simulink model "Sim_Ex32"  (R2022a)
settings: Solver=VariableStepAuto  StartTime=0.0  StopTime=Stop_Time  MaxStep=100e-6  RelTol=1e-3
values from neighbouring files (symbols this model uses):
  Ts = 1/Fs    (= 5e-05)    [A_Ex32.m]
undefined symbols (not defined in the file or in its folder): DiscIntNeverNeededParam, Grid, PLL
settings Model: SimulationMode=accelerator  Creator=Joonhee  LastModifiedBy=light
settings SolverCC: AlgebraicLoopSolver=TrustRegion
settings DataIOCC: ReturnWorkspaceOutputs=off
settings DebuggingCC: UnconnectedInputMsg=warning  UnconnectedOutputMsg=warning  UnconnectedLineMsg=warning  SFMachineParentedDataDiag=warning  ArithmeticOperatorsInVariantConditions=warning
settings SFSimCC: SimUseLocalCustomCode=off  CustomCodeUndefinedFunction=UseInterfaceOnly
settings RTWCC: RTWUseLocalCustomCode=off
settings CodeAppCC: StateflowObjectComments=on

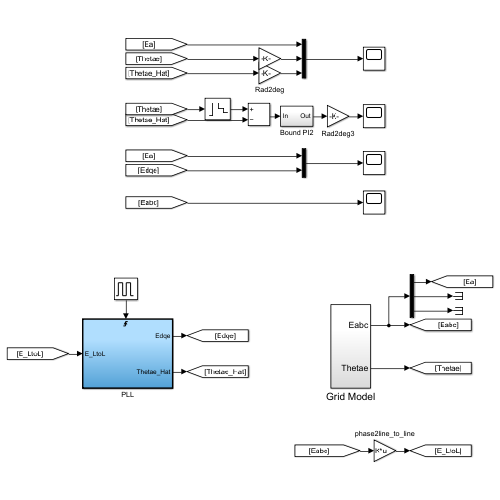
[thumbnail: Simulink's stored preview of the top-level diagram]
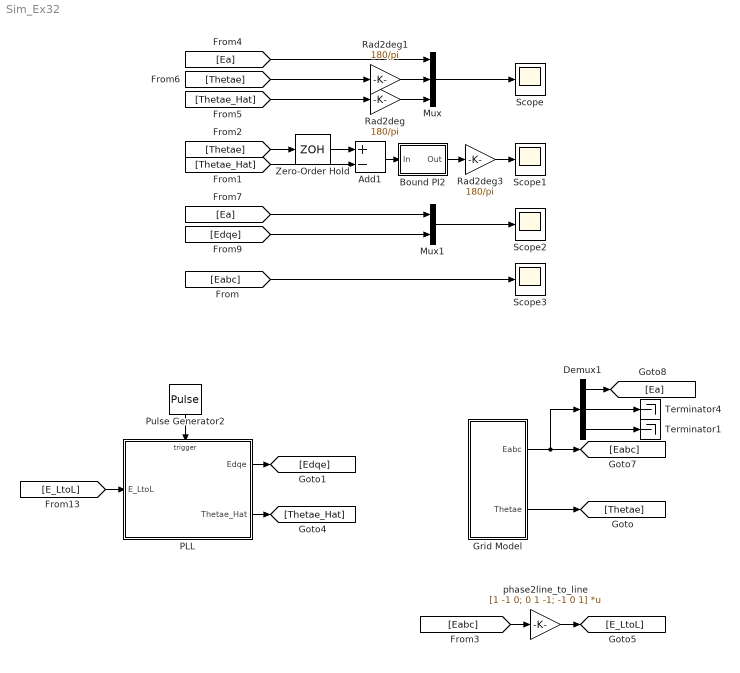
== system Sim_Ex32 ==
  Add1 : Sum  Inputs=+-
  Bound PI2 : Subsystem
  Demux1 : Demux  Outputs=3
  Grid Model : Subsystem
  Mux : Mux  Inputs=3
  Mux1 : Mux  Inputs=2
  PLL : Subsystem  TreatAsAtomicUnit=on
  Pulse Generator2 : DiscretePulseGenerator  PulseType=Time based  Period=Ts  PulseWidth=50
  Rad2deg : Gain  Gain=180/pi
  Rad2deg1 : Gain  Gain=180/pi
  Rad2deg3 : Gain  Gain=180/pi
  Scope{,1..3} (4 alike) : Scope
  Terminator1 : Terminator
  Terminator4 : Terminator
  Zero-Order Hold : ZeroOrderHold  SampleTime=Ts
  phase2line_to_line : Gain  Gain=[1 -1 0; 0 1 -1; -1 0 1]  Multiplication=Matrix(K*u)
  wires:
  Mux/1 -> Scope/1
  [Thetae_Hat] -> Rad2deg/1
  Rad2deg/1 -> Mux/3
  [Thetae] -> Rad2deg1/1
  Rad2deg1/1 -> Mux/2
  [Ea] -> Mux/1
  Mux1/1 -> Scope2/1
  [Ea] -> Mux1/1
  [Edqe] -> Mux1/2
  PLL/2(Thetae_Hat) -> [Thetae_Hat]
  PLL/1(Edqe) -> [Edqe]
  Pulse Generator2/1 -> PLL/Trigger
  Rad2deg3/1 -> Scope1/1
  Add1/1 -> Bound PI2/1(In)
  [Thetae_Hat] -> Add1/2
  Bound PI2/1(Out) -> Rad2deg3/1
  [Thetae] -> Zero-Order Hold/1
  Zero-Order Hold/1 -> Add1/1
  [Eabc] -> Scope3/1
  Demux1/1 -> [Ea]
  Demux1/2 -> Terminator4/1
  Demux1/3 -> Terminator1/1
  phase2line_to_line/1 -> [E_LtoL]
  [Eabc] -> phase2line_to_line/1
  [E_LtoL] -> PLL/1(E_LtoL)
  Grid Model/1(Eabc) -> Demux1/1, [Eabc]
  Grid Model/2(Thetae) -> [Thetae]

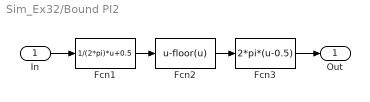
== system Sim_Ex32/Bound PI2 ==
  In : Inport
  Fcn1 : Fcn  Expr=1/(2*pi)*u+0.5
  Fcn2 : Fcn  Expr=u-floor(u)
  Fcn3 : Fcn  Expr=2*pi*(u-0.5)
  Out : Outport
  wires:
  Fcn1/1 -> Fcn2/1
  Fcn2/1 -> Fcn3/1
  In/1 -> Fcn1/1
  Fcn3/1 -> Out/1

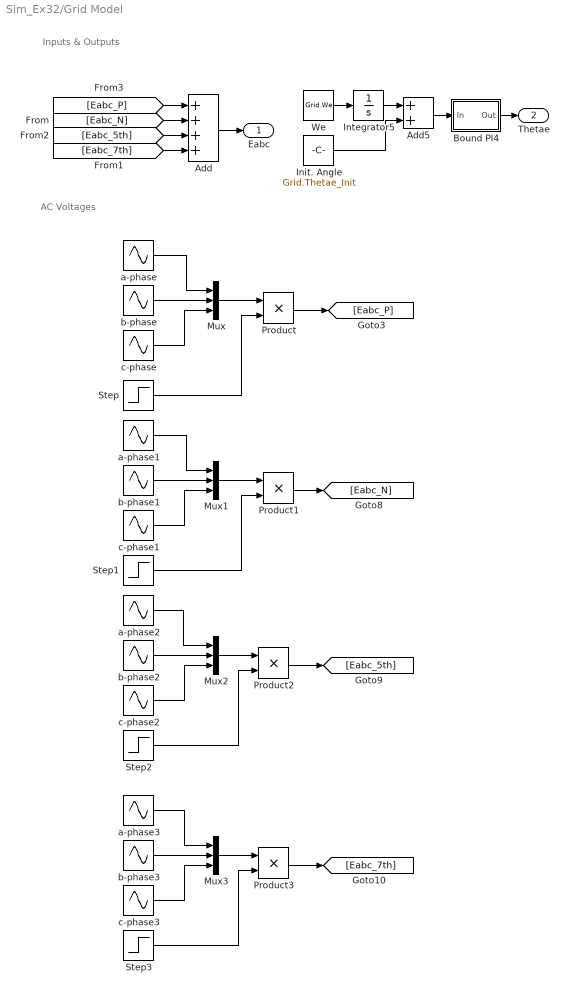
== system Sim_Ex32/Grid Model ==
  note: AC Voltages
  note: Inputs & Outputs
  Add : Sum  Inputs=++++
  Add5 : Sum
  Bound PI4 : Subsystem
  Init. Angle : Constant  Value=Grid.Thetae_Init
  Integrator5 : Integrator
  Mux{,1..3} (4 alike) : Mux  Inputs=3
  Product{,1..3} (4 alike) : Product
  Step : Step  Time=Grid.Time_Fault  Before=1  After=Grid.Ratio_P  SampleTime=0
  Step1 : Step  Time=Grid.Time_Fault  SampleTime=0
  Step2 : Step  Time=Grid.Time_Fault  SampleTime=0
  Step3 : Step  Time=Grid.Time_Fault  SampleTime=0
  We : Constant  Value=Grid.We
  a-phase : Sin  Amplitude=Grid.V_P  Frequency=Grid.We  Phase=Grid.Thetae_Init+pi  SampleTime=0
  a-phase1 : Sin  Amplitude=Grid.V_N  Frequency=Grid.We  Phase=Grid.Thetae_N_Init+pi  SampleTime=0
  a-phase2 : Sin  Amplitude=Grid.V_5th  Frequency=5*Grid.We  Phase=Grid.Thetae_5th_Init+pi  SampleTime=0
  a-phase3 : Sin  Amplitude=Grid.V_7th  Frequency=7*Grid.We  Phase=Grid.Thetae_7th_Init+pi  SampleTime=0
  b-phase : Sin  Amplitude=Grid.V_P  Frequency=Grid.We  Phase=Grid.Thetae_Init+pi-2/3*pi  SampleTime=0
  b-phase1 : Sin  Amplitude=Grid.V_N  Frequency=Grid.We  Phase=Grid.Thetae_N_Init+pi+2/3*pi  SampleTime=0
  b-phase2 : Sin  Amplitude=Grid.V_5th  Frequency=5*Grid.We  Phase=Grid.Thetae_5th_Init+pi+2/3*pi  SampleTime=0
  b-phase3 : Sin  Amplitude=Grid.V_7th  Frequency=7*Grid.We  Phase=Grid.Thetae_7th_Init+pi-2/3*pi  SampleTime=0
  c-phase : Sin  Amplitude=Grid.V_P  Frequency=Grid.We  Phase=Grid.Thetae_Init+pi-4/3*pi  SampleTime=0
  c-phase1 : Sin  Amplitude=Grid.V_N  Frequency=Grid.We  Phase=Grid.Thetae_N_Init+pi+4/3*pi  SampleTime=0
  c-phase2 : Sin  Amplitude=Grid.V_5th  Frequency=5*Grid.We  Phase=Grid.Thetae_5th_Init+pi+4/3*pi  SampleTime=0
  c-phase3 : Sin  Amplitude=Grid.V_7th  Frequency=7*Grid.We  Phase=Grid.Thetae_7th_Init+pi-4/3*pi  SampleTime=0
  Eabc : Outport
  Thetae : Outport  Port=2
  wires:
  [Eabc_P] -> Add/1
  Add/1 -> Eabc/1
  [Eabc_N] -> Add/2
  [Eabc_5th] -> Add/3
  [Eabc_7th] -> Add/4
  Bound PI4/1(Out) -> Thetae/1
  Add5/1 -> Bound PI4/1(In)
  We/1 -> Integrator5/1
  Init. Angle/1 -> Add5/2
  Integrator5/1 -> Add5/1
  b-phase/1 -> Mux/2
  a-phase/1 -> Mux/1
  c-phase/1 -> Mux/3
  c-phase1/1 -> Mux1/3
  a-phase1/1 -> Mux1/1
  b-phase1/1 -> Mux1/2
  b-phase2/1 -> Mux2/2
  a-phase2/1 -> Mux2/1
  c-phase2/1 -> Mux2/3
  c-phase3/1 -> Mux3/3
  a-phase3/1 -> Mux3/1
  b-phase3/1 -> Mux3/2
  Mux/1 -> Product/1
  Mux1/1 -> Product1/1
  Step/1 -> Product/2
  Product/1 -> [Eabc_P]
  Step1/1 -> Product1/2
  Mux2/1 -> Product2/1
  Mux3/1 -> Product3/1
  Step2/1 -> Product2/2
  Step3/1 -> Product3/2
  Product1/1 -> [Eabc_N]
  Product2/1 -> [Eabc_5th]
  Product3/1 -> [Eabc_7th]

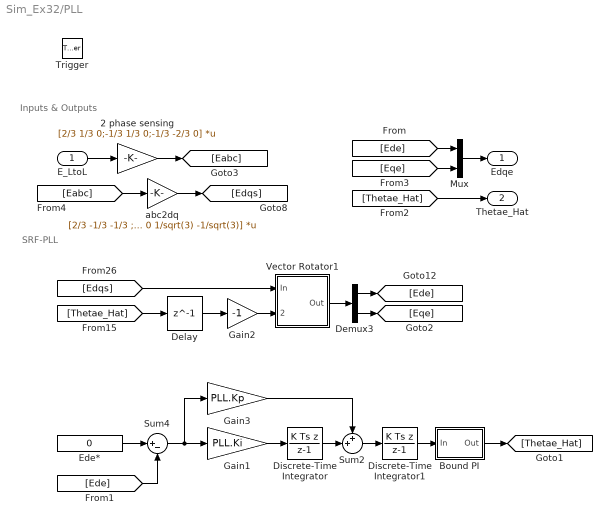
== system Sim_Ex32/PLL ==
  note: Inputs & Outputs
  note: SRF-PLL
  E_LtoL : Inport
  Trigger : TriggerPort  VariantControl=Variant
  2 phase sensing : Gain  Gain=[2/3 1/3 0;-1/3 1/3 0;-1/3 -2/3 0]  Multiplication=Matrix(K*u)  SaturateOnIntegerOverflow=on  OutDataTypeStr=Inherit: Same as input  ParamDataTypeStr=Inherit: Same as input
  Bound PI : Subsystem
  Delay : Delay  DelayLength=1
  Demux3 : Demux  Outputs=2
  Discrete-Time Integrator : DiscreteIntegrator  IntegratorMethod=Integration: Backward Euler  InitialCondition=PLL.We_FF  SampleTime=-1  ICPrevOutput=DiscIntNeverNeededParam  ICPrevScaledInput=DiscIntNeverNeededParam
  Discrete-Time Integrator1 : DiscreteIntegrator  IntegratorMethod=Integration: Backward Euler  InitialCondition=2*Grid.We*Ts  SampleTime=-1  ICPrevOutput=DiscIntNeverNeededParam  ICPrevScaledInput=DiscIntNeverNeededParam
  Ede* : Constant  Value=0
  Gain1 : Gain  Gain=PLL.Ki
  Gain2 : Gain  Gain=-1
  Gain3 : Gain  Gain=PLL.Kp
  Mux : Mux  Inputs=2
  Sum2 : Sum  Inputs=++|
  Sum4 : Sum  Inputs=|+-
  Vector Rotator1 : Subsystem  Tag=dqs2dqw
  abc2dq : Gain  Gain=[2/3 -1/3 -1/3 ; 0 1/sqrt(3) -1/sqrt(3)]  Multiplication=Matrix(K*u)  SaturateOnIntegerOverflow=on  OutDataTypeStr=Inherit: Same as input  ParamDataTypeStr=Inherit: Same as input
  Edqe : Outport
  Thetae_Hat : Outport  Port=2
  wires:
  Discrete-Time Integrator1/1 -> Bound PI/1(In)
  Ede*/1 -> Sum4/1
  Gain1/1 -> Discrete-Time Integrator/1
  [Thetae_Hat] -> Thetae_Hat/1
  Mux/1 -> Edqe/1
  [Edqs] -> Vector Rotator1/1(In)
  [Eabc] -> abc2dq/1
  Sum2/1 -> Discrete-Time Integrator1/1
  Gain3/1 -> Sum2/1
  Vector Rotator1/1(Out) -> Demux3/1
  Bound PI/1(Out) -> [Thetae_Hat]
  abc2dq/1 -> [Edqs]
  Demux3/1 -> [Ede]
  Discrete-Time Integrator/1 -> Sum2/2
  Sum4/1 -> Gain3/1, Gain1/1
  [Ede] -> Sum4/2
  Gain2/1 -> Vector Rotator1/2(Theta)
  [Thetae_Hat] -> Delay/1
  Demux3/2 -> [Eqe]
  [Ede] -> Mux/1
  [Eqe] -> Mux/2
  Delay/1 -> Gain2/1
  2 phase sensing/1 -> [Eabc]
  E_LtoL/1 -> 2 phase sensing/1

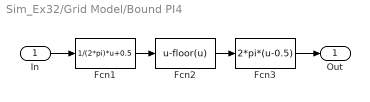
== system Sim_Ex32/Grid Model/Bound PI4 ==
  In : Inport
  Fcn1 : Fcn  Expr=1/(2*pi)*u+0.5
  Fcn2 : Fcn  Expr=u-floor(u)
  Fcn3 : Fcn  Expr=2*pi*(u-0.5)
  Out : Outport
  wires:
  Fcn1/1 -> Fcn2/1
  Fcn2/1 -> Fcn3/1
  In/1 -> Fcn1/1
  Fcn3/1 -> Out/1

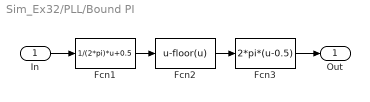
== system Sim_Ex32/PLL/Bound PI ==
  In : Inport
  Fcn1 : Fcn  Expr=1/(2*pi)*u+0.5
  Fcn2 : Fcn  Expr=u-floor(u)
  Fcn3 : Fcn  Expr=2*pi*(u-0.5)
  Out : Outport
  wires:
  Fcn1/1 -> Fcn2/1
  Fcn2/1 -> Fcn3/1
  In/1 -> Fcn1/1
  Fcn3/1 -> Out/1

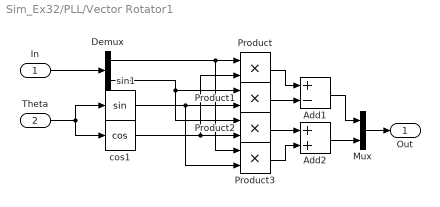
== system Sim_Ex32/PLL/Vector Rotator1 ==
  In : Inport
  Theta : Inport  Port=2
  Add1 : Sum  Inputs=+-
  Add2 : Sum
  Demux : Demux  Outputs=2
  Mux : Mux  Inputs=[1 1]
  Product{,1..3} (4 alike) : Product  RndMeth=Zero
  cos1 : Trigonometry  Operator=cos
  sin1 : Trigonometry
  Out : Outport
  wires:
  Theta/1 -> cos1/1, sin1/1
  Demux/1 -> Product3/1, Product/1
  Mux/1 -> Out/1
  In/1 -> Demux/1
  Demux/2 -> Product1/1, Product2/1
  cos1/1 -> Product/2, Product2/2
  sin1/1 -> Product1/2, Product3/2
  Product/1 -> Add1/1
  Product1/1 -> Add1/2
  Add1/1 -> Mux/1
  Product2/1 -> Add2/1
  Product3/1 -> Add2/2
  Add2/1 -> Mux/2
